simulink model "kalman_filter_test"  (R2025b)
settings: Solver=VariableStepAuto  StartTime=0.0  StopTime=10  RelTol=1e-3  EnableMultiTasking=on
InitFcn:
  | ts = prepareLogForParameterEstimation("../LOGS/log0168.csv")
libraries: simulink x1
settings Model: ModifiedByFormat=The MathWorks Inc.  Creator=The MathWorks, Inc.  LastModifiedBy=The MathWorks Inc.
settings SolverCC: AlgebraicLoopSolver=TrustRegion  AutoInsertRateTranBlk=on
settings DataIOCC: LimitDataPoints=on  SaveFormat=Array  SaveOutput=off  SaveTime=off  ReturnWorkspaceOutputs=off
settings OptimizationCC: DefaultUnderspecifiedDataType=single  ExpressionDepthLimit=2147483647.0  LifeSpan=1
settings DebuggingCC: UnderspecifiedInitializationDetection=Classic  MergeDetectMultiDrivingBlocksExec=none  SolverPrmCheckMsg=warning  FcnCallInpInsideContextMsg=warning  UnconnectedInputMsg=warning  UnconnectedOutputMsg=warning  UnconnectedLineMsg=warning  StateNameClashWarn=warning  SFUnexpectedBacktrackingDiag=warning  SFNoUnconditionalDefaultTransitionDiag=warning  SFExecutionAtInitializationDiag=none  ArithmeticOperatorsInVariantConditions=warning
settings HardwareCC: ProdBitPerPointer=32.0  ProdBitPerSizeT=32.0  ProdBitPerPtrDiffT=32.0  ProdLargestAtomicFloat=None  ProdIntDivRoundTo=Undefined  ProdEndianess=Unspecified  ProdWordSize=32.0  ProdHWDeviceType=32-bit Generic
settings ModelReferenceCC: PropagateSignalLabelsOutOfModel=off
settings SFSimCC: SimUseLocalCustomCode=off  CustomCodeUndefinedFunction=UseInterfaceOnly
settings RTWCC: RTWUseLocalCustomCode=off  GPUComputeCapability=3.5
settings CodeAppCC: StateflowObjectComments=on
settings GRTTargetCC: TargetLangStandard=C89/C90 (ANSI)  CombineOutputUpdateFcns=off  GRTInterface=on
settings ConfigComp: CovMetricSettings=dw  CovSaveCumulativeToWorkspaceVar=on  CovSaveSingleToWorkspaceVar=on  CovExternalEMLEnable=off  CovSFcnEnable=off

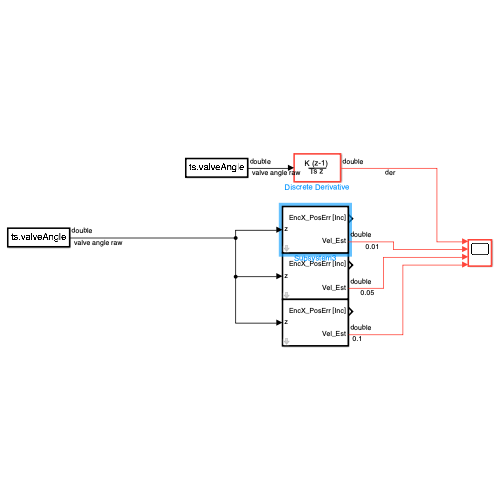
[thumbnail: Simulink's stored preview of the top-level diagram]
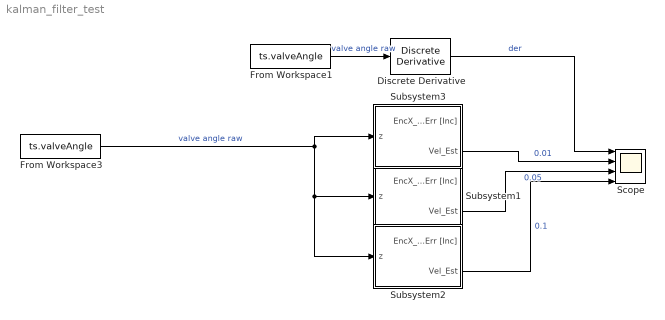
== system kalman_filter_test ==
  Discrete Derivative : simulink/Discrete/Discrete Derivative  gainval=1.0  ICPrevScaledInput=0.0  OutMin=[]  OutMax=[]  OutDataType=fixdt(1, 16)  OutScaling=2^-10  DoSatur=off
  From Workspace1 : FromWorkspace  VariableName=ts.valveAngle  Interpolate=off  OutputAfterFinalValue=Holding final value
  From Workspace3 : FromWorkspace  VariableName=ts.valveAngle  Interpolate=off  OutputAfterFinalValue=Holding final value
  Scope : Scope  NumInputPorts=4
      settings: ActiveDisplayYMinimum=2466.2089195631324  ActiveDisplayYMaximum=3336.8434884020035
  Subsystem1 : Subsystem  mask{Ts=1/4000, lambda_RQ=0.05}
  Subsystem2 : Subsystem  mask{Ts=1/4000, lambda_RQ=0.1}
  Subsystem3 : Subsystem  mask{Ts=1/4000, lambda_RQ=0.01}
  wires:
  From Workspace3/1 -> Subsystem3/1(z), Subsystem2/1(z), Subsystem1/1(z)  "valve angle raw"
  Subsystem3/2(Vel_Est) -> Scope/2  "0.01"
  Subsystem1/2(Vel_Est) -> Scope/3  "0.05"
  Subsystem2/2(Vel_Est) -> Scope/4  "0.1"
  From Workspace1/1 -> Discrete Derivative/1  "valve angle raw"
  Discrete Derivative/1 -> Scope/1  "der"

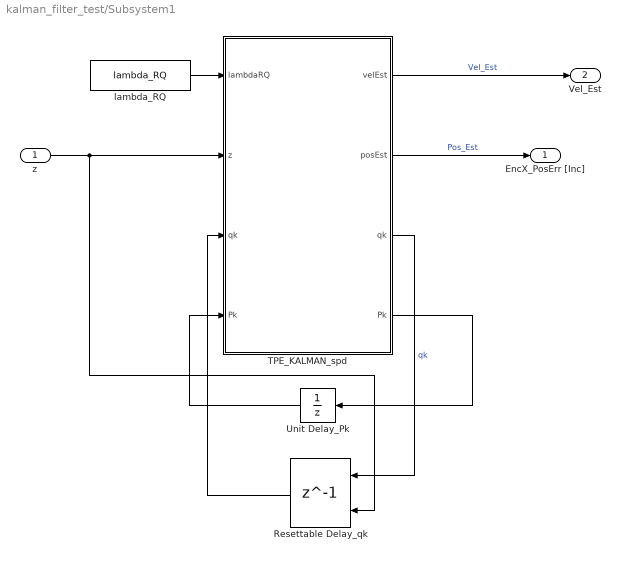
== system kalman_filter_test/Subsystem1 ==
  z : Inport  Unit=deg  PortDimensions=1
  Resettable Delay_qk : Delay  DelayLength=1  InitialConditionSource=Input port  SampleTime=Ts
      settings: InputPortMap=u0,p4
  TPE_KALMAN_spd : MATLAB Function  TreatAsAtomicUnit=on
  Unit Delay_Pk : UnitDelay  InitialCondition=[0.155 65; 65 5.7e4]  SampleTime=Ts  HasFrameUpgradeWarning=on
  lambda_RQ : Constant  Value=lambda_RQ  OutDataTypeStr=double
  EncX_PosErr [Inc] : Outport  OutDataTypeStr=double  Unit=deg  PortDimensions=1  SampleTime=Ts  VectorParamsAs1DForOutWhenUnconnected=off
  Vel_Est : Outport  Port=2  OutDataTypeStr=double  Unit=deg/s  PortDimensions=1  SampleTime=Ts  VectorParamsAs1DForOutWhenUnconnected=off
  wires:
  TPE_KALMAN_spd/4(Pk) -> Unit Delay_Pk/1
  TPE_KALMAN_spd/2(posEst) -> EncX_PosErr [Inc]/1  "Pos_Est"
  TPE_KALMAN_spd/1(velEst) -> Vel_Est/1  "Vel_Est"
  z/1 -> Resettable Delay_qk/2, TPE_KALMAN_spd/2(z)
  TPE_KALMAN_spd/3(qk) -> Resettable Delay_qk/1  "qk"
  lambda_RQ/1 -> TPE_KALMAN_spd/1(lambdaRQ)
  Unit Delay_Pk/1 -> TPE_KALMAN_spd/4("Pk ")
  Resettable Delay_qk/1 -> TPE_KALMAN_spd/3("qk ")

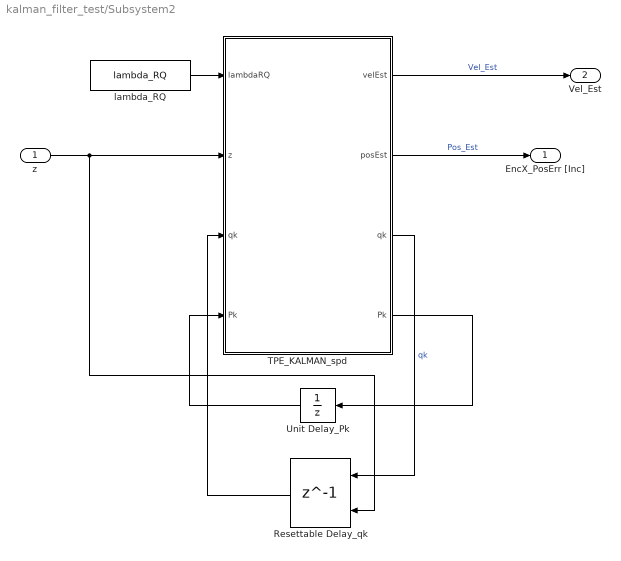
== system kalman_filter_test/Subsystem2 ==
  z : Inport  Unit=deg  PortDimensions=1
  Resettable Delay_qk : Delay  DelayLength=1  InitialConditionSource=Input port  SampleTime=Ts
      settings: InputPortMap=u0,p4
  TPE_KALMAN_spd : MATLAB Function  TreatAsAtomicUnit=on
  Unit Delay_Pk : UnitDelay  InitialCondition=[0.155 65; 65 5.7e4]  SampleTime=Ts  HasFrameUpgradeWarning=on
  lambda_RQ : Constant  Value=lambda_RQ  OutDataTypeStr=double
  EncX_PosErr [Inc] : Outport  OutDataTypeStr=double  Unit=deg  PortDimensions=1  SampleTime=Ts  VectorParamsAs1DForOutWhenUnconnected=off
  Vel_Est : Outport  Port=2  OutDataTypeStr=double  Unit=deg/s  PortDimensions=1  SampleTime=Ts  VectorParamsAs1DForOutWhenUnconnected=off
  wires:
  Resettable Delay_qk/1 -> TPE_KALMAN_spd/3("qk ")
  Unit Delay_Pk/1 -> TPE_KALMAN_spd/4("Pk ")
  lambda_RQ/1 -> TPE_KALMAN_spd/1(lambdaRQ)
  TPE_KALMAN_spd/3(qk) -> Resettable Delay_qk/1  "qk"
  z/1 -> TPE_KALMAN_spd/2(z), Resettable Delay_qk/2
  TPE_KALMAN_spd/1(velEst) -> Vel_Est/1  "Vel_Est"
  TPE_KALMAN_spd/2(posEst) -> EncX_PosErr [Inc]/1  "Pos_Est"
  TPE_KALMAN_spd/4(Pk) -> Unit Delay_Pk/1

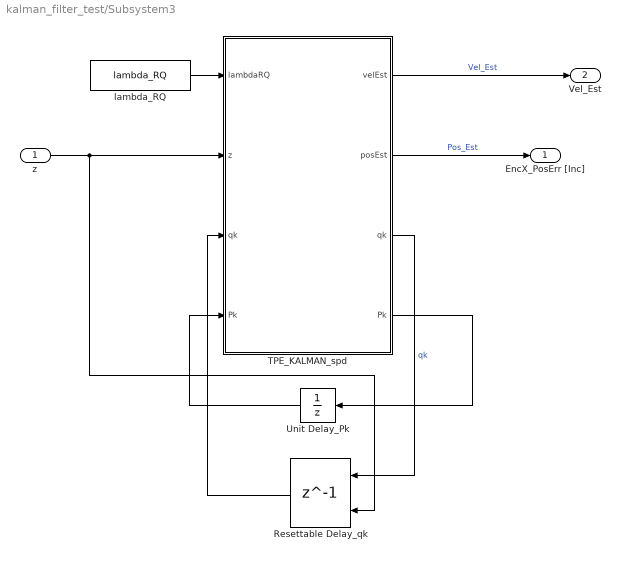
== system kalman_filter_test/Subsystem3 ==
  z : Inport  Unit=deg  PortDimensions=1
  Resettable Delay_qk : Delay  DelayLength=1  InitialConditionSource=Input port  SampleTime=Ts
      settings: InputPortMap=u0,p4
  TPE_KALMAN_spd : MATLAB Function  TreatAsAtomicUnit=on
  Unit Delay_Pk : UnitDelay  InitialCondition=[0.155 65; 65 5.7e4]  SampleTime=Ts  HasFrameUpgradeWarning=on
  lambda_RQ : Constant  Value=lambda_RQ  OutDataTypeStr=double
  EncX_PosErr [Inc] : Outport  OutDataTypeStr=double  Unit=deg  PortDimensions=1  SampleTime=Ts  VectorParamsAs1DForOutWhenUnconnected=off
  Vel_Est : Outport  Port=2  OutDataTypeStr=double  Unit=deg/s  PortDimensions=1  SampleTime=Ts  VectorParamsAs1DForOutWhenUnconnected=off
  wires:
  Resettable Delay_qk/1 -> TPE_KALMAN_spd/3("qk ")
  Unit Delay_Pk/1 -> TPE_KALMAN_spd/4("Pk ")
  lambda_RQ/1 -> TPE_KALMAN_spd/1(lambdaRQ)
  TPE_KALMAN_spd/3(qk) -> Resettable Delay_qk/1  "qk"
  z/1 -> TPE_KALMAN_spd/2(z), Resettable Delay_qk/2
  TPE_KALMAN_spd/1(velEst) -> Vel_Est/1  "Vel_Est"
  TPE_KALMAN_spd/2(posEst) -> EncX_PosErr [Inc]/1  "Pos_Est"
  TPE_KALMAN_spd/4(Pk) -> Unit Delay_Pk/1

== matlab function kalman_filter_test/Subsystem1/TPE_KALMAN_spd ==
  settings: updateMethod=DISCRETE  sampleTime=Ts
  data z settings: description=since it reads the encoder data its made uint32
  data: lambdaRQ input double size=1; velEst output double size=1; posEst output double size=1; qk output size=[2,1]; z input double size=1; qk input double size=[2,1]; Pk input double size=[2,2]; Ts parameter double size=1; Pk output size=[2,2]
function [ velEst, posEst, qk,Pk] =Kalman_X_Enc(lambdaRQ,z, qk, Pk, Ts)
%   200814 
%   --------
% INPUTS
%  z: measurement (1,1) %    [increment]
%   q1: previous state [2Nx1]
%   P1: previous error cov matrix [2Nx2N]
%   qk1: previous state [2x1]
%   Pk1: previous error cov matrix [2x2]
%   nSpindle : Spindle Speed [rpm]
%   IncrSec: increment per second
% PARAMETERS Periodic component
%   Ts      : Sampling time [ms]
%   Q :  process noise covariance matrix [2x2], tunable
%   R  :  measurement noise cov 1x1, tunable

%   R olcerdeki hataa,
%   Q modeldeki hata, Q kuculurse modele guvenir, smooth olur. Ama aynı isi
%   disaridan lambdaRQ carpani ile yapabilirsin.
R_Enc=(360/65536)^2;
Q_Enc=[Ts^3/3, Ts^2/2; Ts^2/2, Ts]*(4/Ts)^2*1e-3;% <<<<<< BUNLA OYNA 1-4-10

%%  Remove the trend with kinematic Kalman Filter
Q=lambdaRQ*Q_Enc;
[qk,Pk] = Kalman_Kinematic(z, qk, Pk, R_Enc,Q,Ts);
velEst = qk(2);%[incr/sec]
posEst=qk(1);


end



function [q,P] = Kalman_Kinematic(z, q, P, R,Q,Ts)
%   First Eqn : Priori state est
PosPrior = q(1)+q(2)*Ts;
VelPrior =q(2);
%   Second Eqn : Priori cov matrix
dummy = P(2,1)+Ts*P(2,2);
P11 = P(1,1)+Ts*P(1,2) + Ts*dummy +Q(1,1);
P21 = dummy+Q(2,1);
P12 = P(1,2)+Ts*P(2,2)+Q(1,2);
P22 = P(2,2)+Q(2,2);

%   Kalman Gain
dummy = 1/(P11+R);
K1= P11*dummy;
K2= P21*dummy; % No need since there is no vel estimate

% State estimate
dummy=z-PosPrior;
q = [PosPrior + K1*dummy;...
    VelPrior+K2*dummy];

%   Covariance Matrix
P=[P11-K1*P11, P12-K1*P12;...
    P21-K2*P11, P22-K2*P12];
end

== matlab function kalman_filter_test/Subsystem2/TPE_KALMAN_spd ==
  settings: updateMethod=DISCRETE  sampleTime=Ts
  data z settings: description=since it reads the encoder data its made uint32
  data: lambdaRQ input double size=1; velEst output double size=1; posEst output double size=1; qk output size=[2,1]; z input double size=1; qk input double size=[2,1]; Pk input double size=[2,2]; Ts parameter double size=1; Pk output size=[2,2]
function [ velEst, posEst, qk,Pk] =Kalman_X_Enc(lambdaRQ,z, qk, Pk, Ts)
%   200814 
%   --------
% INPUTS
%  z: measurement (1,1) %    [increment]
%   q1: previous state [2Nx1]
%   P1: previous error cov matrix [2Nx2N]
%   qk1: previous state [2x1]
%   Pk1: previous error cov matrix [2x2]
%   nSpindle : Spindle Speed [rpm]
%   IncrSec: increment per second
% PARAMETERS Periodic component
%   Ts      : Sampling time [ms]
%   Q :  process noise covariance matrix [2x2], tunable
%   R  :  measurement noise cov 1x1, tunable

%   R olcerdeki hataa,
%   Q modeldeki hata, Q kuculurse modele guvenir, smooth olur. Ama aynı isi
%   disaridan lambdaRQ carpani ile yapabilirsin.
R_Enc=(360/65536)^2;
Q_Enc=[Ts^3/3, Ts^2/2; Ts^2/2, Ts]*(4/Ts)^2*1e-3;% <<<<<< BUNLA OYNA 1-4-10

%%  Remove the trend with kinematic Kalman Filter
Q=lambdaRQ*Q_Enc;
[qk,Pk] = Kalman_Kinematic(z, qk, Pk, R_Enc,Q,Ts);
velEst = qk(2);%[incr/sec]
posEst=qk(1);


end



function [q,P] = Kalman_Kinematic(z, q, P, R,Q,Ts)
%   First Eqn : Priori state est
PosPrior = q(1)+q(2)*Ts;
VelPrior =q(2);
%   Second Eqn : Priori cov matrix
dummy = P(2,1)+Ts*P(2,2);
P11 = P(1,1)+Ts*P(1,2) + Ts*dummy +Q(1,1);
P21 = dummy+Q(2,1);
P12 = P(1,2)+Ts*P(2,2)+Q(1,2);
P22 = P(2,2)+Q(2,2);

%   Kalman Gain
dummy = 1/(P11+R);
K1= P11*dummy;
K2= P21*dummy; % No need since there is no vel estimate

% State estimate
dummy=z-PosPrior;
q = [PosPrior + K1*dummy;...
    VelPrior+K2*dummy];

%   Covariance Matrix
P=[P11-K1*P11, P12-K1*P12;...
    P21-K2*P11, P22-K2*P12];
end

== matlab function kalman_filter_test/Subsystem3/TPE_KALMAN_spd ==
  settings: updateMethod=DISCRETE  sampleTime=Ts
  data z settings: description=since it reads the encoder data its made uint32
  data: lambdaRQ input double size=1; velEst output double size=1; posEst output double size=1; qk output size=[2,1]; z input double size=1; qk input double size=[2,1]; Pk input double size=[2,2]; Ts parameter double size=1; Pk output size=[2,2]
function [ velEst, posEst, qk,Pk] =Kalman_X_Enc(lambdaRQ,z, qk, Pk, Ts)
%   200814 
%   --------
% INPUTS
%  z: measurement (1,1) %    [increment]
%   q1: previous state [2Nx1]
%   P1: previous error cov matrix [2Nx2N]
%   qk1: previous state [2x1]
%   Pk1: previous error cov matrix [2x2]
%   nSpindle : Spindle Speed [rpm]
%   IncrSec: increment per second
% PARAMETERS Periodic component
%   Ts      : Sampling time [ms]
%   Q :  process noise covariance matrix [2x2], tunable
%   R  :  measurement noise cov 1x1, tunable

%   R olcerdeki hataa,
%   Q modeldeki hata, Q kuculurse modele guvenir, smooth olur. Ama aynı isi
%   disaridan lambdaRQ carpani ile yapabilirsin.
R_Enc=(360/65536)^2;
Q_Enc=[Ts^3/3, Ts^2/2; Ts^2/2, Ts]*(4/Ts)^2*1e-3;% <<<<<< BUNLA OYNA 1-4-10

%%  Remove the trend with kinematic Kalman Filter
Q=lambdaRQ*Q_Enc;
[qk,Pk] = Kalman_Kinematic(z, qk, Pk, R_Enc,Q,Ts);
velEst = qk(2);%[incr/sec]
posEst=qk(1);


end



function [q,P] = Kalman_Kinematic(z, q, P, R,Q,Ts)
%   First Eqn : Priori state est
PosPrior = q(1)+q(2)*Ts;
VelPrior =q(2);
%   Second Eqn : Priori cov matrix
dummy = P(2,1)+Ts*P(2,2);
P11 = P(1,1)+Ts*P(1,2) + Ts*dummy +Q(1,1);
P21 = dummy+Q(2,1);
P12 = P(1,2)+Ts*P(2,2)+Q(1,2);
P22 = P(2,2)+Q(2,2);

%   Kalman Gain
dummy = 1/(P11+R);
K1= P11*dummy;
K2= P21*dummy; % No need since there is no vel estimate

% State estimate
dummy=z-PosPrior;
q = [PosPrior + K1*dummy;...
    VelPrior+K2*dummy];

%   Covariance Matrix
P=[P11-K1*P11, P12-K1*P12;...
    P21-K2*P11, P22-K2*P12];
end
